simulink model "closedLoop_tuned"  (R2019a)
settings: Solver=ode14x  StartTime=0.0  StopTime=20  FixedStep=ts  RelTol=1e-3
undefined symbols (not defined in the file): ts
libraries: simulink x12, controlLibrary x12, mechLibrary x1
CloseFcn:
  | try,close(h1_elec_motor_brushless_dc),end
  | clear h1_elec_motor_brushless_dc
  | 
  | clear simlog_elec_motor_brushless_dc
  | clear logsout_elec_motor_brushless_dc
  | 
  | 
  | clear tout
Description:
  | Position feedback control, with servomotors, of a robot arm. Controllers are discretised.
  | 
  | Copyright 2008-2019 The MathWorks, Inc.
settings Model: DataDictionary=robotDataDictionary.sldd  EnableAccessToBaseWorkspace=off  Creator=MathWorks  LastModifiedBy=falderis
settings ConfigSet: Description=Configuration set for closed loop system
settings SolverCC: ExtrapolationOrder=1  SolverJacobianMethodControl=SparsePerturbation  AutoInsertRateTranBlk=on
settings DataIOCC: SaveFormat=StructureWithTime  SaveOutput=off  ReturnWorkspaceOutputsName=simulationOutput
settings OptimizationCC: BlockReduction=off  DefaultParameterBehavior=Inlined  EnhancedBackFolding=on  PassReuseOutputArgsAs=Individual arguments  OptimizeBlockOrder=speed  DifferentSizesBufferReuse=on  OptimizationCustomize=off
settings DebuggingCC: ParameterTunabilityLossMsg=error  BusObjectLabelMismatch=error  SFUnexpectedBacktrackingDiag=warning  SFNoUnconditionalDefaultTransitionDiag=warning  SFExecutionAtInitializationDiag=none  ArithmeticOperatorsInVariantConditions=warning
settings HardwareCC: ProdBitPerPointer=32  ProdBitPerSizeT=32  ProdBitPerPtrDiffT=32  ProdLargestAtomicFloat=None  ProdWordSize=32  ProdLongLongMode=on  ProdHWDeviceType=Generic->32-bit x86 compatible
settings ModelReferenceCC: ModelReferenceNumInstancesAllowed=Single  PropagateSignalLabelsOutOfModel=off
settings SFSimCC: SimUseLocalCustomCode=off  MATLABDynamicMemAlloc=off
settings RTWCC: SystemTargetFile=ert.tlc  TemplateMakefile=ert_default_tmf  GenerateReport=on  RTWVerbose=off  RTWUseLocalCustomCode=off  IncludeHyperlinkInReport=on  LaunchReport=on  CodeExecutionProfiling=on  GenerateTraceInfo=on  GenerateTraceReport=on  GenerateTraceReportSl=on  GenerateTraceReportSf=on  GenerateTraceReportEml=on  RTWCompilerOptimization=on
settings CodeAppCC: ForceParamTrailComments=on  IgnoreCustomStorageClasses=off  OperatorAnnotations=on  SimulinkDataObjDesc=on  SFDataObjDesc=on  InsertBlockDesc=on
settings ERTTargetCC: GenerateSampleERTMain=on  InlinedParameterPlacement=NonHierarchical  ERTCustomFileTemplate=example_file_process.tlc
settings ConfigComp: CovMetricSettings=dw  CovHtmlReporting=on  CovSaveCumulativeToWorkspaceVar=on  CovSaveSingleToWorkspaceVar=on  CovExternalEMLEnable=off  CovSFcnEnable=off
settings SimscapeCC: SimscapeNormalizeSystem=off  SimscapeLogName=mechPlant_simlog  SimscapeLogLimitData=off
settings ConfigurationSet: Description=SimMechanics 2G
settings ExplorerConfigSet: InternalSimMechanicsExplorerSettings="<ExplorerConfiguration><canonicalview>planar_xy</canonicalview><AnimationSetting><BasePlaybackSpeed>1.0</BasePlaybackSpeed><PlaybackSpeedFactor>1.0</PlaybackSpeedFactor></AnimationSetting><TilePanel><TileInfo><Tiles Columns=\"1\" Count=\"1\" Rows=\"1\"><Column Left=\"2\" Weight=\"1\"/><Column Left=\"833\"/><Row Top=\"2\" Weight=\"1\"/><Row Top=\"616\"/><Tile Height=\"1\" Width=\"1\" X=\"0\" Y=\"0\"/></Tiles></TileInfo><SceneInfo><SceneViewer><BGColor><R>0.60000002384185791</R><G>0.60000002384185791</G><B>0.60000002384185791</B></BGColor><Camera><Position><X>0.40313583982721529</X><Y>0.401665542364257</Y><Z>0.3417126092405493</Z></Position><Center><X>0.080205141109062281</X><Y>0.078734843646070099</Y><Z>0.018781910522366958</Z></Center><Up><X>-0.40824829046386307</X><Y>0.81649658092772615</Y><Z>-0.40824829046386307</Z></Up><Left>-0.31441769609555942</Left><Right>0.31441769609555942</Right><Bottom>-0.27755873043819368</Bottom><Top>0.27755873043819368</Top></Camera></SceneViewer></SceneInfo></TilePanel></ExplorerConfiguration>"

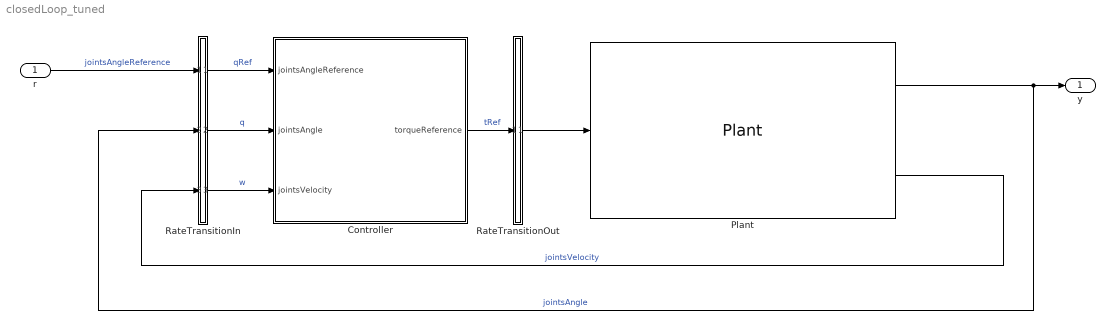
== system closedLoop_tuned ==
  r : Inport  OutDataTypeStr=Bus: jointMotionBus  Unit=deg  SampleTime=0
  Controller : Subsystem
      mask Display: image('controller.png')
  Plant : mechLibrary/Plant  SystemSampleTime=-1
  RateTransitionIn : Subsystem
  RateTransitionOut : Subsystem
  y : Outport  OutDataTypeStr=Bus: jointMotionBus  Unit=deg
  wires:
  Controller/1(torqueReference) -> RateTransitionOut/1(tRefIn)  "tRef"
  RateTransitionIn/1(qRef) -> Controller/1(jointsAngleReference)  "qRef"
  Plant/2 -> RateTransitionIn/3(wIn)  "jointsVelocity"
  RateTransitionOut/1(tRef) -> Plant/1
  RateTransitionIn/3(w) -> Controller/3(jointsVelocity)  "w"
  Plant/1 -> y/1, RateTransitionIn/2(qIn)  "jointsAngle"
  r/1 -> RateTransitionIn/1(qRefIn)  "jointsAngleReference"
  RateTransitionIn/2(q) -> Controller/2(jointsAngle)  "q"

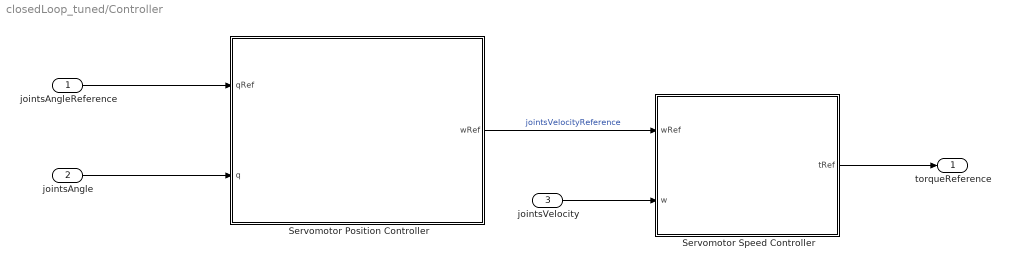
== system closedLoop_tuned/Controller ==
  jointsAngleReference : Inport  OutDataTypeStr=Bus: jointMotionBus  Unit=deg  SampleTime=ts
  jointsAngle : Inport  Port=2  OutDataTypeStr=Bus: jointMotionBus  Unit=deg  SampleTime=ts
  jointsVelocity : Inport  Port=3  OutDataTypeStr=Bus: jointVelBus  Unit=deg/s  SampleTime=ts
  Servomotor Position Controller : Subsystem  VariantControl=SV
      mask Display: image('pid.png');
  Servomotor Speed Controller : Subsystem
      mask Display: image('pi2.png');
  torqueReference : Outport  OutDataTypeStr=Bus: jointTorqueBus  Unit=N*m  SampleTime=ts
  wires:
  jointsAngle/1 -> Servomotor Position Controller/2(q)
  jointsAngleReference/1 -> Servomotor Position Controller/1(qRef)
  Servomotor Speed Controller/1(tRef) -> torqueReference/1
  Servomotor Position Controller/1(wRef) -> Servomotor Speed Controller/1(wRef)  "jointsVelocityReference"
  jointsVelocity/1 -> Servomotor Speed Controller/2(w)

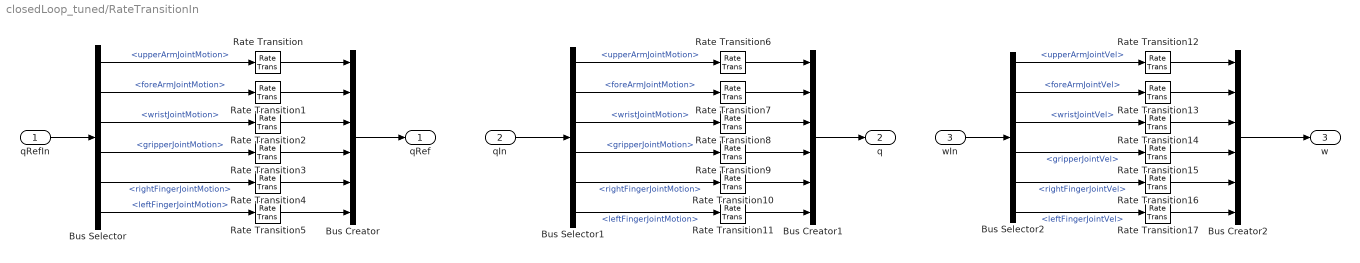
== system closedLoop_tuned/RateTransitionIn ==
  qRefIn : Inport  OutDataTypeStr=Bus: jointMotionBus  Unit=deg
  qIn : Inport  Port=2  OutDataTypeStr=Bus: jointMotionBus  Unit=deg
  wIn : Inport  Port=3  OutDataTypeStr=Bus: jointVelBus
  Bus Creator : BusCreator  Inputs=6  OutDataTypeStr=Bus: jointMotionBus
      settings: InheritFromInputs=off
  Bus Creator1 : BusCreator  Inputs=6  OutDataTypeStr=Bus: jointMotionBus
      settings: InheritFromInputs=off
  Bus Creator2 : BusCreator  Inputs=6  OutDataTypeStr=Bus: jointVelBus
      settings: InheritFromInputs=off
  Bus Selector : BusSelector  OutputSignals=upperArmJointMotion,foreArmJointMotion,wristJointMotion,gripperJointMotion,rightFingerJointMotion,leftFingerJointMotion
  Bus Selector1 : BusSelector  OutputSignals=upperArmJointMotion,foreArmJointMotion,wristJointMotion,gripperJointMotion,rightFingerJointMotion,leftFingerJointMotion
  Bus Selector2 : BusSelector  OutputSignals=upperArmJointVel,foreArmJointVel,wristJointVel,gripperJointVel,rightFingerJointVel,leftFingerJointVel
  Rate Transition{,1..17} (18 alike) : RateTransition  OutPortSampleTime=ts
  qRef : Outport  OutDataTypeStr=Bus: jointMotionBus
  q : Outport  Port=2  OutDataTypeStr=Bus: jointMotionBus
  w : Outport  Port=3  OutDataTypeStr=Bus: jointVelBus
  wires:
  Bus Selector1/6 -> Rate Transition11/1  "<leftFingerJointMotion>"
  Bus Selector1/3 -> Rate Transition8/1  "<wristJointMotion>"
  qIn/1 -> Bus Selector1/1
  Bus Selector1/1 -> Rate Transition6/1  "<upperArmJointMotion>"
  Bus Selector1/5 -> Rate Transition10/1  "<rightFingerJointMotion>"
  Bus Selector/6 -> Rate Transition5/1  "<leftFingerJointMotion>"
  Bus Selector1/4 -> Rate Transition9/1  "<gripperJointMotion>"
  Bus Selector/2 -> Rate Transition1/1  "<foreArmJointMotion>"
  Bus Selector1/2 -> Rate Transition7/1  "<foreArmJointMotion>"
  Bus Selector/3 -> Rate Transition2/1  "<wristJointMotion>"
  Bus Selector/4 -> Rate Transition3/1  "<gripperJointMotion>"
  Bus Selector/1 -> Rate Transition/1  "<upperArmJointMotion>"
  qRefIn/1 -> Bus Selector/1
  Bus Selector/5 -> Rate Transition4/1  "<rightFingerJointMotion>"
  Bus Selector2/5 -> Rate Transition16/1  "<rightFingerJointVel>"
  Bus Selector2/4 -> Rate Transition15/1  "<gripperJointVel>"
  Bus Selector2/3 -> Rate Transition14/1  "<wristJointVel>"
  wIn/1 -> Bus Selector2/1
  Bus Selector2/1 -> Rate Transition12/1  "<upperArmJointVel>"
  Bus Selector2/2 -> Rate Transition13/1  "<foreArmJointVel>"
  Bus Selector2/6 -> Rate Transition17/1  "<leftFingerJointVel>"
  Rate Transition/1 -> Bus Creator/1
  Rate Transition1/1 -> Bus Creator/2
  Rate Transition2/1 -> Bus Creator/3
  Rate Transition3/1 -> Bus Creator/4
  Rate Transition4/1 -> Bus Creator/5
  Rate Transition5/1 -> Bus Creator/6
  Bus Creator/1 -> qRef/1
  Rate Transition7/1 -> Bus Creator1/2
  Rate Transition11/1 -> Bus Creator1/6
  Bus Creator1/1 -> q/1
  Rate Transition9/1 -> Bus Creator1/4
  Rate Transition6/1 -> Bus Creator1/1
  Rate Transition8/1 -> Bus Creator1/3
  Rate Transition10/1 -> Bus Creator1/5
  Rate Transition12/1 -> Bus Creator2/1
  Rate Transition13/1 -> Bus Creator2/2
  Rate Transition14/1 -> Bus Creator2/3
  Rate Transition15/1 -> Bus Creator2/4
  Rate Transition16/1 -> Bus Creator2/5
  Rate Transition17/1 -> Bus Creator2/6
  Bus Creator2/1 -> w/1

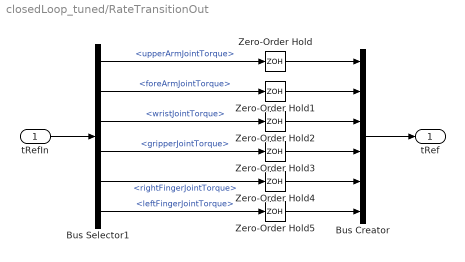
== system closedLoop_tuned/RateTransitionOut ==
  tRefIn : Inport  OutDataTypeStr=Bus: jointTorqueBus  Unit=N*m
  Bus Creator : BusCreator  Inputs=6  OutDataTypeStr=Bus: jointTorqueBus
      settings: InheritFromInputs=off
  Bus Selector1 : BusSelector  OutputSignals=upperArmJointTorque,foreArmJointTorque,wristJointTorque,gripperJointTorque,rightFingerJointTorque,leftFingerJointTorque
  Zero-Order Hold{,1..5} (6 alike) : ZeroOrderHold  SampleTime=-1
  tRef : Outport  OutDataTypeStr=Bus: jointTorqueBus  SampleTime=0
  wires:
  Bus Selector1/3 -> Zero-Order Hold2/1  "<wristJointTorque>"
  tRefIn/1 -> Bus Selector1/1
  Bus Selector1/2 -> Zero-Order Hold1/1  "<foreArmJointTorque>"
  Bus Selector1/5 -> Zero-Order Hold4/1  "<rightFingerJointTorque>"
  Bus Selector1/4 -> Zero-Order Hold3/1  "<gripperJointTorque>"
  Bus Selector1/1 -> Zero-Order Hold/1  "<upperArmJointTorque>"
  Bus Selector1/6 -> Zero-Order Hold5/1  "<leftFingerJointTorque>"
  Zero-Order Hold5/1 -> Bus Creator/6
  Zero-Order Hold4/1 -> Bus Creator/5
  Zero-Order Hold1/1 -> Bus Creator/2
  Zero-Order Hold/1 -> Bus Creator/1
  Zero-Order Hold2/1 -> Bus Creator/3
  Zero-Order Hold3/1 -> Bus Creator/4
  Bus Creator/1 -> tRef/1

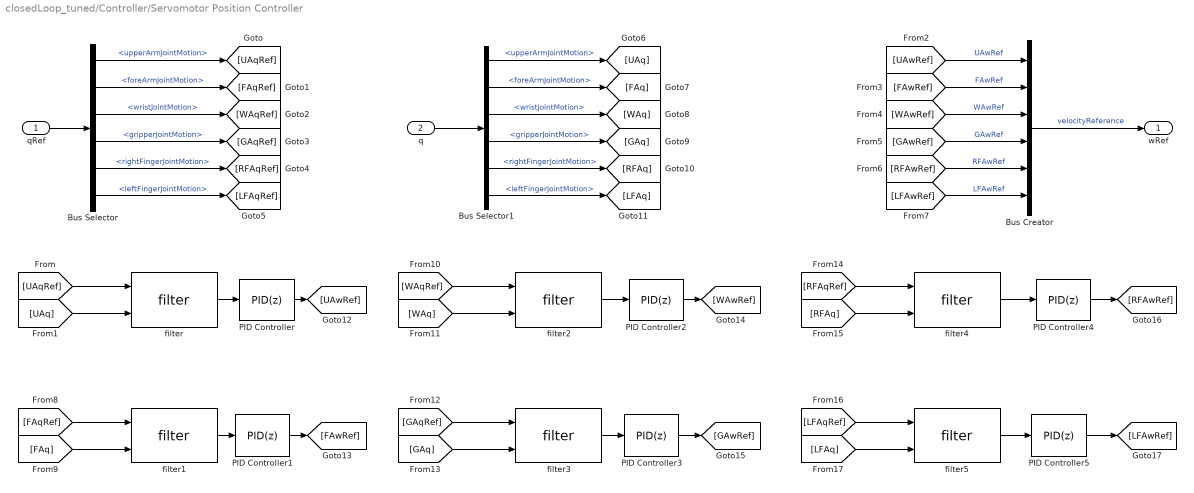
== system closedLoop_tuned/Controller/Servomotor Position Controller ==
  qRef : Inport  OutDataTypeStr=Bus: jointMotionBus  Unit=deg
  q : Inport  Port=2  OutDataTypeStr=Bus: jointMotionBus  Unit=deg
  Bus Creator : BusCreator  Inputs=6  OutDataTypeStr=Bus: jointVelBus
      settings: InheritFromInputs=off
  Bus Selector : BusSelector  OutputSignals=upperArmJointMotion,foreArmJointMotion,wristJointMotion,gripperJointMotion,rightFingerJointMotion,leftFingerJointMotion
  Bus Selector1 : BusSelector  OutputSignals=upperArmJointMotion,foreArmJointMotion,wristJointMotion,gripperJointMotion,rightFingerJointMotion,leftFingerJointMotion
  PID Controller : simulink/Continuous/PID Controller  Controller=PID  Form=Parallel  TimeDomain=Discrete-time  SampleTime=ts  IntegratorMethod=Forward Euler  FilterMethod=Forward Euler  ControllerParametersSource=internal  P=10.4708336285486  I=0.000419222702982036  D=0.346600752490046  UseFilter=on  N=761.904761904762  TunerSelectOption=Transfer Function Based (PID Tuner App)  InitialConditionSource=internal  InitialConditionForIntegrator=0  InitialConditionForFilter=0  DifferentiatorICPrevScaledInput=0  ExternalReset=none  TrackingMode=off  Kt=1  LimitOutput=off  UpperSaturationLimit=inf  LowerSaturationLimit=-inf  LinearizeAsGain=on  AntiWindupMode=none  Kb=1  POutMin=[]  POutMax=[]  IOutMin=[]  IOutMax=[]  DOutMin=[]  DOutMax=[]  NOutMin=[]  NOutMax=[]  SumOutMin=[]  SumOutMax=[]  SaturationOutMin=[]  SaturationOutMax=[]  PParamMin=[]  PParamMax=[]  IParamMin=[]  IParamMax=[]  DParamMin=[]  DParamMax=[]  NParamMin=[]  NParamMax=[]  KbParamMin=[]  KbParamMax=[]  KtParamMin=[]  KtParamMax=[]  KbOutMin=[]  KbOutMax=[]  KtOutMin=[]  KtOutMax=[]  IntegratorOutMin=[]  IntegratorOutMax=[]  FilterOutMin=[]  FilterOutMax=[]  SumI1OutMin=[]  SumI1OutMax=[]  SumI2OutMin=[]  SumI2OutMax=[]  SumI3OutMin=[]  SumI3OutMax=[]  SumI4OutMin=[]  SumI4OutMax=[]  SumDOutMin=[]  SumDOutMax=[]  DifferentiatorOutMin=[]  DifferentiatorOutMax=[]  FilterDiffOutCoefMin=[]  FilterDiffOutCoefMax=[]  ReciprocalOutMin=[]  ReciprocalOutMax=[]  SumDenOutMin=[]  SumDenOutMax=[]  SumNumOutMin=[]  SumNumOutMax=[]  DivideOutMin=[]  DivideOutMax=[]  IntegratorContinuousStateAttributes=''  IntegratorStateMustResolveToSignalObject=off  IntegratorRTWStateStorageClass=Auto  FilterContinuousStateAttributes=''  FilterStateMustResolveToSignalObject=off  FilterRTWStateStorageClass=Auto  ParallelPVariant=InternalParameters  IdealPVariant=Disabled  IVariant=InternalParameters  DVariant=InternalParameters  IntegratorVariant=Discrete  SatVariant=Disabled  AWVariant=Passthrough  PCopyVariant=Disabled  TRVariant=Disabled  FdbkBlocksVariant=Forward  IdealPFdbkVariant=Disabled  SatFdbkVariant=Disabled  DerivativeFilterVariant=ForwardEulerFilter  NVariant=InternalParameters  NCopyVariant=Disabled  FilterICVariant=InternalICsFilter  IntegratorICVariant=InternalICs  ExternalResetVariant=Disabled  TRSumVariant=Passthrough  SumFdbkVariant=Disabled  SumVariant=Sum_PID
  PID Controller1 : simulink/Continuous/PID Controller  Controller=PID  Form=Parallel  TimeDomain=Discrete-time  SampleTime=ts  IntegratorMethod=Forward Euler  FilterMethod=Forward Euler  ControllerParametersSource=internal  P=10.7694124560307  I=0.000593032145468798  D=21.0180234727249  UseFilter=on  N=4.00240654506278e-05  TunerSelectOption=Transfer Function Based (PID Tuner App)  InitialConditionSource=internal  InitialConditionForIntegrator=0  InitialConditionForFilter=0  DifferentiatorICPrevScaledInput=0  ExternalReset=none  TrackingMode=off  Kt=1  LimitOutput=off  UpperSaturationLimit=inf  LowerSaturationLimit=-inf  LinearizeAsGain=on  AntiWindupMode=none  Kb=1  POutMin=[]  POutMax=[]  IOutMin=[]  IOutMax=[]  DOutMin=[]  DOutMax=[]  NOutMin=[]  NOutMax=[]  SumOutMin=[]  SumOutMax=[]  SaturationOutMin=[]  SaturationOutMax=[]  PParamMin=[]  PParamMax=[]  IParamMin=[]  IParamMax=[]  DParamMin=[]  DParamMax=[]  NParamMin=[]  NParamMax=[]  KbParamMin=[]  KbParamMax=[]  KtParamMin=[]  KtParamMax=[]  KbOutMin=[]  KbOutMax=[]  KtOutMin=[]  KtOutMax=[]  IntegratorOutMin=[]  IntegratorOutMax=[]  FilterOutMin=[]  FilterOutMax=[]  SumI1OutMin=[]  SumI1OutMax=[]  SumI2OutMin=[]  SumI2OutMax=[]  SumI3OutMin=[]  SumI3OutMax=[]  SumI4OutMin=[]  SumI4OutMax=[]  SumDOutMin=[]  SumDOutMax=[]  DifferentiatorOutMin=[]  DifferentiatorOutMax=[]  FilterDiffOutCoefMin=[]  FilterDiffOutCoefMax=[]  ReciprocalOutMin=[]  ReciprocalOutMax=[]  SumDenOutMin=[]  SumDenOutMax=[]  SumNumOutMin=[]  SumNumOutMax=[]  DivideOutMin=[]  DivideOutMax=[]  IntegratorContinuousStateAttributes=''  IntegratorStateMustResolveToSignalObject=off  IntegratorRTWStateStorageClass=Auto  FilterContinuousStateAttributes=''  FilterStateMustResolveToSignalObject=off  FilterRTWStateStorageClass=Auto  ParallelPVariant=InternalParameters  IdealPVariant=Disabled  IVariant=InternalParameters  DVariant=InternalParameters  IntegratorVariant=Discrete  SatVariant=Disabled  AWVariant=Passthrough  PCopyVariant=Disabled  TRVariant=Disabled  FdbkBlocksVariant=Forward  IdealPFdbkVariant=Disabled  SatFdbkVariant=Disabled  DerivativeFilterVariant=ForwardEulerFilter  NVariant=InternalParameters  NCopyVariant=Disabled  FilterICVariant=InternalICsFilter  IntegratorICVariant=InternalICs  ExternalResetVariant=Disabled  TRSumVariant=Passthrough  SumFdbkVariant=Disabled  SumVariant=Sum_PID
  PID Controller2 : simulink/Continuous/PID Controller  Controller=PID  Form=Parallel  TimeDomain=Discrete-time  SampleTime=ts  IntegratorMethod=Forward Euler  FilterMethod=Forward Euler  ControllerParametersSource=internal  P=10.8442867281081  I=0.000448190430142682  D=0.223470955257761  UseFilter=on  N=761.904761904762  TunerSelectOption=Transfer Function Based (PID Tuner App)  InitialConditionSource=internal  InitialConditionForIntegrator=0  InitialConditionForFilter=0  DifferentiatorICPrevScaledInput=0  ExternalReset=none  TrackingMode=off  Kt=1  LimitOutput=off  UpperSaturationLimit=inf  LowerSaturationLimit=-inf  LinearizeAsGain=on  AntiWindupMode=none  Kb=1  POutMin=[]  POutMax=[]  IOutMin=[]  IOutMax=[]  DOutMin=[]  DOutMax=[]  NOutMin=[]  NOutMax=[]  SumOutMin=[]  SumOutMax=[]  SaturationOutMin=[]  SaturationOutMax=[]  PParamMin=[]  PParamMax=[]  IParamMin=[]  IParamMax=[]  DParamMin=[]  DParamMax=[]  NParamMin=[]  NParamMax=[]  KbParamMin=[]  KbParamMax=[]  KtParamMin=[]  KtParamMax=[]  KbOutMin=[]  KbOutMax=[]  KtOutMin=[]  KtOutMax=[]  IntegratorOutMin=[]  IntegratorOutMax=[]  FilterOutMin=[]  FilterOutMax=[]  SumI1OutMin=[]  SumI1OutMax=[]  SumI2OutMin=[]  SumI2OutMax=[]  SumI3OutMin=[]  SumI3OutMax=[]  SumI4OutMin=[]  SumI4OutMax=[]  SumDOutMin=[]  SumDOutMax=[]  DifferentiatorOutMin=[]  DifferentiatorOutMax=[]  FilterDiffOutCoefMin=[]  FilterDiffOutCoefMax=[]  ReciprocalOutMin=[]  ReciprocalOutMax=[]  SumDenOutMin=[]  SumDenOutMax=[]  SumNumOutMin=[]  SumNumOutMax=[]  DivideOutMin=[]  DivideOutMax=[]  IntegratorContinuousStateAttributes=''  IntegratorStateMustResolveToSignalObject=off  IntegratorRTWStateStorageClass=Auto  FilterContinuousStateAttributes=''  FilterStateMustResolveToSignalObject=off  FilterRTWStateStorageClass=Auto  ParallelPVariant=InternalParameters  IdealPVariant=Disabled  IVariant=InternalParameters  DVariant=InternalParameters  IntegratorVariant=Discrete  SatVariant=Disabled  AWVariant=Passthrough  PCopyVariant=Disabled  TRVariant=Disabled  FdbkBlocksVariant=Forward  IdealPFdbkVariant=Disabled  SatFdbkVariant=Disabled  DerivativeFilterVariant=ForwardEulerFilter  NVariant=InternalParameters  NCopyVariant=Disabled  FilterICVariant=InternalICsFilter  IntegratorICVariant=InternalICs  ExternalResetVariant=Disabled  TRSumVariant=Passthrough  SumFdbkVariant=Disabled  SumVariant=Sum_PID
  PID Controller3 : simulink/Continuous/PID Controller  Controller=PID  Form=Parallel  TimeDomain=Discrete-time  SampleTime=ts  IntegratorMethod=Forward Euler  FilterMethod=Forward Euler  ControllerParametersSource=internal  P=9.66802754702183  I=0.000444755466308859  D=58.2762205966547  UseFilter=on  N=0.0216415897548656  TunerSelectOption=Transfer Function Based (PID Tuner App)  InitialConditionSource=internal  InitialConditionForIntegrator=0  InitialConditionForFilter=0  DifferentiatorICPrevScaledInput=0  ExternalReset=none  TrackingMode=off  Kt=1  LimitOutput=off  UpperSaturationLimit=inf  LowerSaturationLimit=-inf  LinearizeAsGain=on  AntiWindupMode=none  Kb=1  POutMin=[]  POutMax=[]  IOutMin=[]  IOutMax=[]  DOutMin=[]  DOutMax=[]  NOutMin=[]  NOutMax=[]  SumOutMin=[]  SumOutMax=[]  SaturationOutMin=[]  SaturationOutMax=[]  PParamMin=[]  PParamMax=[]  IParamMin=[]  IParamMax=[]  DParamMin=[]  DParamMax=[]  NParamMin=[]  NParamMax=[]  KbParamMin=[]  KbParamMax=[]  KtParamMin=[]  KtParamMax=[]  KbOutMin=[]  KbOutMax=[]  KtOutMin=[]  KtOutMax=[]  IntegratorOutMin=[]  IntegratorOutMax=[]  FilterOutMin=[]  FilterOutMax=[]  SumI1OutMin=[]  SumI1OutMax=[]  SumI2OutMin=[]  SumI2OutMax=[]  SumI3OutMin=[]  SumI3OutMax=[]  SumI4OutMin=[]  SumI4OutMax=[]  SumDOutMin=[]  SumDOutMax=[]  DifferentiatorOutMin=[]  DifferentiatorOutMax=[]  FilterDiffOutCoefMin=[]  FilterDiffOutCoefMax=[]  ReciprocalOutMin=[]  ReciprocalOutMax=[]  SumDenOutMin=[]  SumDenOutMax=[]  SumNumOutMin=[]  SumNumOutMax=[]  DivideOutMin=[]  DivideOutMax=[]  IntegratorContinuousStateAttributes=''  IntegratorStateMustResolveToSignalObject=off  IntegratorRTWStateStorageClass=Auto  FilterContinuousStateAttributes=''  FilterStateMustResolveToSignalObject=off  FilterRTWStateStorageClass=Auto  ParallelPVariant=InternalParameters  IdealPVariant=Disabled  IVariant=InternalParameters  DVariant=InternalParameters  IntegratorVariant=Discrete  SatVariant=Disabled  AWVariant=Passthrough  PCopyVariant=Disabled  TRVariant=Disabled  FdbkBlocksVariant=Forward  IdealPFdbkVariant=Disabled  SatFdbkVariant=Disabled  DerivativeFilterVariant=ForwardEulerFilter  NVariant=InternalParameters  NCopyVariant=Disabled  FilterICVariant=InternalICsFilter  IntegratorICVariant=InternalICs  ExternalResetVariant=Disabled  TRSumVariant=Passthrough  SumFdbkVariant=Disabled  SumVariant=Sum_PID
  PID Controller4 : simulink/Continuous/PID Controller  Controller=PID  Form=Parallel  TimeDomain=Discrete-time  SampleTime=ts  IntegratorMethod=Forward Euler  FilterMethod=Forward Euler  ControllerParametersSource=internal  P=10.7702769040942  I=0.00097597573827831  D=0.195709489924621  UseFilter=on  N=190.172011630327  TunerSelectOption=Transfer Function Based (PID Tuner App)  InitialConditionSource=internal  InitialConditionForIntegrator=0  InitialConditionForFilter=0  DifferentiatorICPrevScaledInput=0  ExternalReset=none  TrackingMode=off  Kt=1  LimitOutput=off  UpperSaturationLimit=inf  LowerSaturationLimit=-inf  LinearizeAsGain=on  AntiWindupMode=none  Kb=1  POutMin=[]  POutMax=[]  IOutMin=[]  IOutMax=[]  DOutMin=[]  DOutMax=[]  NOutMin=[]  NOutMax=[]  SumOutMin=[]  SumOutMax=[]  SaturationOutMin=[]  SaturationOutMax=[]  PParamMin=[]  PParamMax=[]  IParamMin=[]  IParamMax=[]  DParamMin=[]  DParamMax=[]  NParamMin=[]  NParamMax=[]  KbParamMin=[]  KbParamMax=[]  KtParamMin=[]  KtParamMax=[]  KbOutMin=[]  KbOutMax=[]  KtOutMin=[]  KtOutMax=[]  IntegratorOutMin=[]  IntegratorOutMax=[]  FilterOutMin=[]  FilterOutMax=[]  SumI1OutMin=[]  SumI1OutMax=[]  SumI2OutMin=[]  SumI2OutMax=[]  SumI3OutMin=[]  SumI3OutMax=[]  SumI4OutMin=[]  SumI4OutMax=[]  SumDOutMin=[]  SumDOutMax=[]  DifferentiatorOutMin=[]  DifferentiatorOutMax=[]  FilterDiffOutCoefMin=[]  FilterDiffOutCoefMax=[]  ReciprocalOutMin=[]  ReciprocalOutMax=[]  SumDenOutMin=[]  SumDenOutMax=[]  SumNumOutMin=[]  SumNumOutMax=[]  DivideOutMin=[]  DivideOutMax=[]  IntegratorContinuousStateAttributes=''  IntegratorStateMustResolveToSignalObject=off  IntegratorRTWStateStorageClass=Auto  FilterContinuousStateAttributes=''  FilterStateMustResolveToSignalObject=off  FilterRTWStateStorageClass=Auto  ParallelPVariant=InternalParameters  IdealPVariant=Disabled  IVariant=InternalParameters  DVariant=InternalParameters  IntegratorVariant=Discrete  SatVariant=Disabled  AWVariant=Passthrough  PCopyVariant=Disabled  TRVariant=Disabled  FdbkBlocksVariant=Forward  IdealPFdbkVariant=Disabled  SatFdbkVariant=Disabled  DerivativeFilterVariant=ForwardEulerFilter  NVariant=InternalParameters  NCopyVariant=Disabled  FilterICVariant=InternalICsFilter  IntegratorICVariant=InternalICs  ExternalResetVariant=Disabled  TRSumVariant=Passthrough  SumFdbkVariant=Disabled  SumVariant=Sum_PID
  PID Controller5 : simulink/Continuous/PID Controller  Controller=PID  Form=Parallel  TimeDomain=Discrete-time  SampleTime=ts  IntegratorMethod=Forward Euler  FilterMethod=Forward Euler  ControllerParametersSource=internal  P=10.7654470599538  I=0.00114163073091871  D=0.20047626148189  UseFilter=on  N=257.755378801474  TunerSelectOption=Transfer Function Based (PID Tuner App)  InitialConditionSource=internal  InitialConditionForIntegrator=0  InitialConditionForFilter=0  DifferentiatorICPrevScaledInput=0  ExternalReset=none  TrackingMode=off  Kt=1  LimitOutput=off  UpperSaturationLimit=inf  LowerSaturationLimit=-inf  LinearizeAsGain=on  AntiWindupMode=none  Kb=1  POutMin=[]  POutMax=[]  IOutMin=[]  IOutMax=[]  DOutMin=[]  DOutMax=[]  NOutMin=[]  NOutMax=[]  SumOutMin=[]  SumOutMax=[]  SaturationOutMin=[]  SaturationOutMax=[]  PParamMin=[]  PParamMax=[]  IParamMin=[]  IParamMax=[]  DParamMin=[]  DParamMax=[]  NParamMin=[]  NParamMax=[]  KbParamMin=[]  KbParamMax=[]  KtParamMin=[]  KtParamMax=[]  KbOutMin=[]  KbOutMax=[]  KtOutMin=[]  KtOutMax=[]  IntegratorOutMin=[]  IntegratorOutMax=[]  FilterOutMin=[]  FilterOutMax=[]  SumI1OutMin=[]  SumI1OutMax=[]  SumI2OutMin=[]  SumI2OutMax=[]  SumI3OutMin=[]  SumI3OutMax=[]  SumI4OutMin=[]  SumI4OutMax=[]  SumDOutMin=[]  SumDOutMax=[]  DifferentiatorOutMin=[]  DifferentiatorOutMax=[]  FilterDiffOutCoefMin=[]  FilterDiffOutCoefMax=[]  ReciprocalOutMin=[]  ReciprocalOutMax=[]  SumDenOutMin=[]  SumDenOutMax=[]  SumNumOutMin=[]  SumNumOutMax=[]  DivideOutMin=[]  DivideOutMax=[]  IntegratorContinuousStateAttributes=''  IntegratorStateMustResolveToSignalObject=off  IntegratorRTWStateStorageClass=Auto  FilterContinuousStateAttributes=''  FilterStateMustResolveToSignalObject=off  FilterRTWStateStorageClass=Auto  ParallelPVariant=InternalParameters  IdealPVariant=Disabled  IVariant=InternalParameters  DVariant=InternalParameters  IntegratorVariant=Discrete  SatVariant=Disabled  AWVariant=Passthrough  PCopyVariant=Disabled  TRVariant=Disabled  FdbkBlocksVariant=Forward  IdealPFdbkVariant=Disabled  SatFdbkVariant=Disabled  DerivativeFilterVariant=ForwardEulerFilter  NVariant=InternalParameters  NCopyVariant=Disabled  FilterICVariant=InternalICsFilter  IntegratorICVariant=InternalICs  ExternalResetVariant=Disabled  TRSumVariant=Passthrough  SumFdbkVariant=Disabled  SumVariant=Sum_PID
  filter{,1..5} (6 alike) : controlLibrary/filter  tc=1e-2  sampleTime=ts
  wRef : Outport  OutDataTypeStr=Bus: jointVelBus  Unit=deg/s
  wires:
  qRef/1 -> Bus Selector/1
  q/1 -> Bus Selector1/1
  Bus Selector/1 -> [UAqRef]  "<upperArmJointMotion>"
  Bus Selector/2 -> [FAqRef]  "<foreArmJointMotion>"
  Bus Selector/3 -> [WAqRef]  "<wristJointMotion>"
  Bus Selector/4 -> [GAqRef]  "<gripperJointMotion>"
  Bus Selector/5 -> [RFAqRef]  "<rightFingerJointMotion>"
  Bus Selector/6 -> [LFAqRef]  "<leftFingerJointMotion>"
  Bus Selector1/1 -> [UAq]  "<upperArmJointMotion>"
  Bus Selector1/3 -> [WAq]  "<wristJointMotion>"
  Bus Selector1/2 -> [FAq]  "<foreArmJointMotion>"
  Bus Selector1/5 -> [RFAq]  "<rightFingerJointMotion>"
  Bus Selector1/4 -> [GAq]  "<gripperJointMotion>"
  Bus Selector1/6 -> [LFAq]  "<leftFingerJointMotion>"
  [UAwRef] -> Bus Creator/1  "UAwRef"
  [FAwRef] -> Bus Creator/2  "FAwRef"
  [WAwRef] -> Bus Creator/3  "WAwRef"
  [GAwRef] -> Bus Creator/4  "GAwRef"
  [RFAwRef] -> Bus Creator/5  "RFAwRef"
  [LFAwRef] -> Bus Creator/6  "LFAwRef"
  Bus Creator/1 -> wRef/1  "velocityReference"
  filter5/1 -> PID Controller5/1
  [RFAq] -> filter4/2
  [LFAq] -> filter5/2
  [FAqRef] -> filter1/1
  [GAqRef] -> filter3/1
  filter3/1 -> PID Controller3/1
  [UAq] -> filter/2
  [RFAqRef] -> filter4/1
  [WAq] -> filter2/2
  [UAqRef] -> filter/1
  filter2/1 -> PID Controller2/1
  [WAqRef] -> filter2/1
  [FAq] -> filter1/2
  [GAq] -> filter3/2
  [LFAqRef] -> filter5/1
  filter4/1 -> PID Controller4/1
  filter/1 -> PID Controller/1
  PID Controller/1 -> [UAwRef]
  PID Controller2/1 -> [WAwRef]
  PID Controller3/1 -> [GAwRef]
  PID Controller4/1 -> [RFAwRef]
  PID Controller5/1 -> [LFAwRef]
  filter1/1 -> PID Controller1/1
  PID Controller1/1 -> [FAwRef]

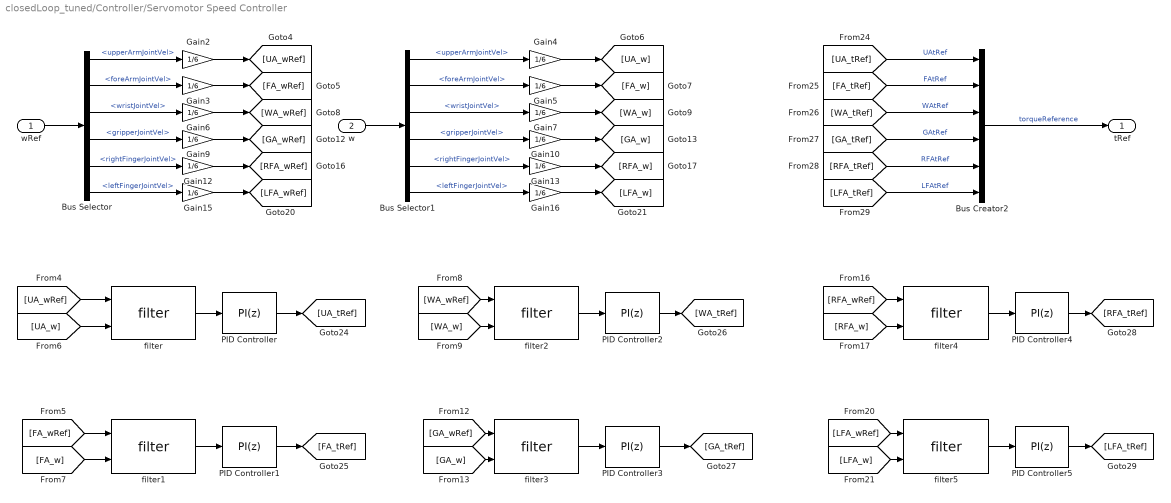
== system closedLoop_tuned/Controller/Servomotor Speed Controller ==
  wRef : Inport  OutDataTypeStr=Bus: jointVelBus
  w : Inport  Port=2  OutDataTypeStr=Bus: jointVelBus
  Bus Creator2 : BusCreator  Inputs=6  OutDataTypeStr=Bus: jointTorqueBus
      settings: InheritFromInputs=off
  Bus Selector : BusSelector  OutputSignals=upperArmJointVel,foreArmJointVel,wristJointVel,gripperJointVel,rightFingerJointVel,leftFingerJointVel
  Bus Selector1 : BusSelector  OutputSignals=upperArmJointVel,foreArmJointVel,wristJointVel,gripperJointVel,rightFingerJointVel,leftFingerJointVel
  Gain{2..7,9..10,12..13,15..16} (12 alike) : Gain  Gain=1/6
  PID Controller : simulink/Continuous/PID Controller  Controller=PI  Form=Parallel  TimeDomain=Discrete-time  SampleTime=ts  IntegratorMethod=Forward Euler  FilterMethod=Forward Euler  ControllerParametersSource=internal  P=0.0360231984902585  I=0.00337174988064101  D=0  UseFilter=on  N=0  TunerSelectOption=Transfer Function Based (PID Tuner App)  InitialConditionSource=internal  InitialConditionForIntegrator=0  InitialConditionForFilter=0  DifferentiatorICPrevScaledInput=0  ExternalReset=none  TrackingMode=off  Kt=1  LimitOutput=off  UpperSaturationLimit=inf  LowerSaturationLimit=-inf  LinearizeAsGain=on  AntiWindupMode=none  Kb=1  POutMin=[]  POutMax=[]  IOutMin=[]  IOutMax=[]  DOutMin=[]  DOutMax=[]  NOutMin=[]  NOutMax=[]  SumOutMin=[]  SumOutMax=[]  SaturationOutMin=[]  SaturationOutMax=[]  PParamMin=[]  PParamMax=[]  IParamMin=[]  IParamMax=[]  DParamMin=[]  DParamMax=[]  NParamMin=[]  NParamMax=[]  KbParamMin=[]  KbParamMax=[]  KtParamMin=[]  KtParamMax=[]  KbOutMin=[]  KbOutMax=[]  KtOutMin=[]  KtOutMax=[]  IntegratorOutMin=[]  IntegratorOutMax=[]  FilterOutMin=[]  FilterOutMax=[]  SumI1OutMin=[]  SumI1OutMax=[]  SumI2OutMin=[]  SumI2OutMax=[]  SumI3OutMin=[]  SumI3OutMax=[]  SumI4OutMin=[]  SumI4OutMax=[]  SumDOutMin=[]  SumDOutMax=[]  DifferentiatorOutMin=[]  DifferentiatorOutMax=[]  FilterDiffOutCoefMin=[]  FilterDiffOutCoefMax=[]  ReciprocalOutMin=[]  ReciprocalOutMax=[]  SumDenOutMin=[]  SumDenOutMax=[]  SumNumOutMin=[]  SumNumOutMax=[]  DivideOutMin=[]  DivideOutMax=[]  IntegratorContinuousStateAttributes=''  IntegratorStateMustResolveToSignalObject=off  IntegratorRTWStateStorageClass=Auto  FilterContinuousStateAttributes=''  FilterStateMustResolveToSignalObject=off  FilterRTWStateStorageClass=Auto  ParallelPVariant=InternalParameters  IdealPVariant=Disabled  IVariant=InternalParameters  DVariant=Disabled  IntegratorVariant=Discrete  SatVariant=Disabled  AWVariant=Passthrough  PCopyVariant=Disabled  TRVariant=Disabled  FdbkBlocksVariant=Forward  IdealPFdbkVariant=Disabled  SatFdbkVariant=Disabled  DerivativeFilterVariant=Disabled  NVariant=Disabled  NCopyVariant=Disabled_SignalSpec  FilterICVariant=Disabled  IntegratorICVariant=InternalICs  ExternalResetVariant=Disabled  TRSumVariant=Passthrough  SumFdbkVariant=Disabled  SumVariant=Sum_PI
  PID Controller1 : simulink/Continuous/PID Controller  Controller=PI  Form=Parallel  TimeDomain=Discrete-time  SampleTime=ts  IntegratorMethod=Forward Euler  FilterMethod=Forward Euler  ControllerParametersSource=internal  P=0.0192799899284329  I=2.06091269945642  D=0  UseFilter=on  N=0  TunerSelectOption=Transfer Function Based (PID Tuner App)  InitialConditionSource=internal  InitialConditionForIntegrator=0  InitialConditionForFilter=0  DifferentiatorICPrevScaledInput=0  ExternalReset=none  TrackingMode=off  Kt=1  LimitOutput=off  UpperSaturationLimit=inf  LowerSaturationLimit=-inf  LinearizeAsGain=on  AntiWindupMode=none  Kb=1  POutMin=[]  POutMax=[]  IOutMin=[]  IOutMax=[]  DOutMin=[]  DOutMax=[]  NOutMin=[]  NOutMax=[]  SumOutMin=[]  SumOutMax=[]  SaturationOutMin=[]  SaturationOutMax=[]  PParamMin=[]  PParamMax=[]  IParamMin=[]  IParamMax=[]  DParamMin=[]  DParamMax=[]  NParamMin=[]  NParamMax=[]  KbParamMin=[]  KbParamMax=[]  KtParamMin=[]  KtParamMax=[]  KbOutMin=[]  KbOutMax=[]  KtOutMin=[]  KtOutMax=[]  IntegratorOutMin=[]  IntegratorOutMax=[]  FilterOutMin=[]  FilterOutMax=[]  SumI1OutMin=[]  SumI1OutMax=[]  SumI2OutMin=[]  SumI2OutMax=[]  SumI3OutMin=[]  SumI3OutMax=[]  SumI4OutMin=[]  SumI4OutMax=[]  SumDOutMin=[]  SumDOutMax=[]  DifferentiatorOutMin=[]  DifferentiatorOutMax=[]  FilterDiffOutCoefMin=[]  FilterDiffOutCoefMax=[]  ReciprocalOutMin=[]  ReciprocalOutMax=[]  SumDenOutMin=[]  SumDenOutMax=[]  SumNumOutMin=[]  SumNumOutMax=[]  DivideOutMin=[]  DivideOutMax=[]  IntegratorContinuousStateAttributes=''  IntegratorStateMustResolveToSignalObject=off  IntegratorRTWStateStorageClass=Auto  FilterContinuousStateAttributes=''  FilterStateMustResolveToSignalObject=off  FilterRTWStateStorageClass=Auto  ParallelPVariant=InternalParameters  IdealPVariant=Disabled  IVariant=InternalParameters  DVariant=Disabled  IntegratorVariant=Discrete  SatVariant=Disabled  AWVariant=Passthrough  PCopyVariant=Disabled  TRVariant=Disabled  FdbkBlocksVariant=Forward  IdealPFdbkVariant=Disabled  SatFdbkVariant=Disabled  DerivativeFilterVariant=Disabled  NVariant=Disabled  NCopyVariant=Disabled_SignalSpec  FilterICVariant=Disabled  IntegratorICVariant=InternalICs  ExternalResetVariant=Disabled  TRSumVariant=Passthrough  SumFdbkVariant=Disabled  SumVariant=Sum_PI
  PID Controller2 : simulink/Continuous/PID Controller  Controller=PI  Form=Parallel  TimeDomain=Discrete-time  SampleTime=ts  IntegratorMethod=Forward Euler  FilterMethod=Forward Euler  ControllerParametersSource=internal  P=0.0426832255455665  I=0.0265288646840578  D=0  UseFilter=on  N=0  TunerSelectOption=Transfer Function Based (PID Tuner App)  InitialConditionSource=internal  InitialConditionForIntegrator=0  InitialConditionForFilter=0  DifferentiatorICPrevScaledInput=0  ExternalReset=none  TrackingMode=off  Kt=1  LimitOutput=off  UpperSaturationLimit=inf  LowerSaturationLimit=-inf  LinearizeAsGain=on  AntiWindupMode=none  Kb=1  POutMin=[]  POutMax=[]  IOutMin=[]  IOutMax=[]  DOutMin=[]  DOutMax=[]  NOutMin=[]  NOutMax=[]  SumOutMin=[]  SumOutMax=[]  SaturationOutMin=[]  SaturationOutMax=[]  PParamMin=[]  PParamMax=[]  IParamMin=[]  IParamMax=[]  DParamMin=[]  DParamMax=[]  NParamMin=[]  NParamMax=[]  KbParamMin=[]  KbParamMax=[]  KtParamMin=[]  KtParamMax=[]  KbOutMin=[]  KbOutMax=[]  KtOutMin=[]  KtOutMax=[]  IntegratorOutMin=[]  IntegratorOutMax=[]  FilterOutMin=[]  FilterOutMax=[]  SumI1OutMin=[]  SumI1OutMax=[]  SumI2OutMin=[]  SumI2OutMax=[]  SumI3OutMin=[]  SumI3OutMax=[]  SumI4OutMin=[]  SumI4OutMax=[]  SumDOutMin=[]  SumDOutMax=[]  DifferentiatorOutMin=[]  DifferentiatorOutMax=[]  FilterDiffOutCoefMin=[]  FilterDiffOutCoefMax=[]  ReciprocalOutMin=[]  ReciprocalOutMax=[]  SumDenOutMin=[]  SumDenOutMax=[]  SumNumOutMin=[]  SumNumOutMax=[]  DivideOutMin=[]  DivideOutMax=[]  IntegratorContinuousStateAttributes=''  IntegratorStateMustResolveToSignalObject=off  IntegratorRTWStateStorageClass=Auto  FilterContinuousStateAttributes=''  FilterStateMustResolveToSignalObject=off  FilterRTWStateStorageClass=Auto  ParallelPVariant=InternalParameters  IdealPVariant=Disabled  IVariant=InternalParameters  DVariant=Disabled  IntegratorVariant=Discrete  SatVariant=Disabled  AWVariant=Passthrough  PCopyVariant=Disabled  TRVariant=Disabled  FdbkBlocksVariant=Forward  IdealPFdbkVariant=Disabled  SatFdbkVariant=Disabled  DerivativeFilterVariant=Disabled  NVariant=Disabled  NCopyVariant=Disabled_SignalSpec  FilterICVariant=Disabled  IntegratorICVariant=InternalICs  ExternalResetVariant=Disabled  TRSumVariant=Passthrough  SumFdbkVariant=Disabled  SumVariant=Sum_PI
  PID Controller3 : simulink/Continuous/PID Controller  Controller=PI  Form=Parallel  TimeDomain=Discrete-time  SampleTime=ts  IntegratorMethod=Forward Euler  FilterMethod=Forward Euler  ControllerParametersSource=internal  P=0.00572339896932079  I=0.460092048608168  D=0  UseFilter=on  N=0  TunerSelectOption=Transfer Function Based (PID Tuner App)  InitialConditionSource=internal  InitialConditionForIntegrator=0  InitialConditionForFilter=0  DifferentiatorICPrevScaledInput=0  ExternalReset=none  TrackingMode=off  Kt=1  LimitOutput=off  UpperSaturationLimit=inf  LowerSaturationLimit=-inf  LinearizeAsGain=on  AntiWindupMode=none  Kb=1  POutMin=[]  POutMax=[]  IOutMin=[]  IOutMax=[]  DOutMin=[]  DOutMax=[]  NOutMin=[]  NOutMax=[]  SumOutMin=[]  SumOutMax=[]  SaturationOutMin=[]  SaturationOutMax=[]  PParamMin=[]  PParamMax=[]  IParamMin=[]  IParamMax=[]  DParamMin=[]  DParamMax=[]  NParamMin=[]  NParamMax=[]  KbParamMin=[]  KbParamMax=[]  KtParamMin=[]  KtParamMax=[]  KbOutMin=[]  KbOutMax=[]  KtOutMin=[]  KtOutMax=[]  IntegratorOutMin=[]  IntegratorOutMax=[]  FilterOutMin=[]  FilterOutMax=[]  SumI1OutMin=[]  SumI1OutMax=[]  SumI2OutMin=[]  SumI2OutMax=[]  SumI3OutMin=[]  SumI3OutMax=[]  SumI4OutMin=[]  SumI4OutMax=[]  SumDOutMin=[]  SumDOutMax=[]  DifferentiatorOutMin=[]  DifferentiatorOutMax=[]  FilterDiffOutCoefMin=[]  FilterDiffOutCoefMax=[]  ReciprocalOutMin=[]  ReciprocalOutMax=[]  SumDenOutMin=[]  SumDenOutMax=[]  SumNumOutMin=[]  SumNumOutMax=[]  DivideOutMin=[]  DivideOutMax=[]  IntegratorContinuousStateAttributes=''  IntegratorStateMustResolveToSignalObject=off  IntegratorRTWStateStorageClass=Auto  FilterContinuousStateAttributes=''  FilterStateMustResolveToSignalObject=off  FilterRTWStateStorageClass=Auto  ParallelPVariant=InternalParameters  IdealPVariant=Disabled  IVariant=InternalParameters  DVariant=Disabled  IntegratorVariant=Discrete  SatVariant=Disabled  AWVariant=Passthrough  PCopyVariant=Disabled  TRVariant=Disabled  FdbkBlocksVariant=Forward  IdealPFdbkVariant=Disabled  SatFdbkVariant=Disabled  DerivativeFilterVariant=Disabled  NVariant=Disabled  NCopyVariant=Disabled_SignalSpec  FilterICVariant=Disabled  IntegratorICVariant=InternalICs  ExternalResetVariant=Disabled  TRSumVariant=Passthrough  SumFdbkVariant=Disabled  SumVariant=Sum_PI
  PID Controller4 : simulink/Continuous/PID Controller  Controller=PI  Form=Parallel  TimeDomain=Discrete-time  SampleTime=ts  IntegratorMethod=Forward Euler  FilterMethod=Forward Euler  ControllerParametersSource=internal  P=0.00659405389444924  I=0.324359106529765  D=0  UseFilter=on  N=0  TunerSelectOption=Transfer Function Based (PID Tuner App)  InitialConditionSource=internal  InitialConditionForIntegrator=0  InitialConditionForFilter=0  DifferentiatorICPrevScaledInput=0  ExternalReset=none  TrackingMode=off  Kt=1  LimitOutput=off  UpperSaturationLimit=0.001  LowerSaturationLimit=-0.001  LinearizeAsGain=on  AntiWindupMode=none  Kb=1  POutMin=[]  POutMax=[]  IOutMin=[]  IOutMax=[]  DOutMin=[]  DOutMax=[]  NOutMin=[]  NOutMax=[]  SumOutMin=[]  SumOutMax=[]  SaturationOutMin=[]  SaturationOutMax=[]  PParamMin=[]  PParamMax=[]  IParamMin=[]  IParamMax=[]  DParamMin=[]  DParamMax=[]  NParamMin=[]  NParamMax=[]  KbParamMin=[]  KbParamMax=[]  KtParamMin=[]  KtParamMax=[]  KbOutMin=[]  KbOutMax=[]  KtOutMin=[]  KtOutMax=[]  IntegratorOutMin=[]  IntegratorOutMax=[]  FilterOutMin=[]  FilterOutMax=[]  SumI1OutMin=[]  SumI1OutMax=[]  SumI2OutMin=[]  SumI2OutMax=[]  SumI3OutMin=[]  SumI3OutMax=[]  SumI4OutMin=[]  SumI4OutMax=[]  SumDOutMin=[]  SumDOutMax=[]  DifferentiatorOutMin=[]  DifferentiatorOutMax=[]  FilterDiffOutCoefMin=[]  FilterDiffOutCoefMax=[]  ReciprocalOutMin=[]  ReciprocalOutMax=[]  SumDenOutMin=[]  SumDenOutMax=[]  SumNumOutMin=[]  SumNumOutMax=[]  DivideOutMin=[]  DivideOutMax=[]  IntegratorContinuousStateAttributes=''  IntegratorStateMustResolveToSignalObject=off  IntegratorRTWStateStorageClass=Auto  FilterContinuousStateAttributes=''  FilterStateMustResolveToSignalObject=off  FilterRTWStateStorageClass=Auto  ParallelPVariant=InternalParameters  IdealPVariant=Disabled  IVariant=InternalParameters  DVariant=Disabled  IntegratorVariant=Discrete  SatVariant=Disabled  AWVariant=Passthrough  PCopyVariant=Disabled  TRVariant=Disabled  FdbkBlocksVariant=Forward  IdealPFdbkVariant=Disabled  SatFdbkVariant=Disabled  DerivativeFilterVariant=Disabled  NVariant=Disabled  NCopyVariant=Disabled_SignalSpec  FilterICVariant=Disabled  IntegratorICVariant=InternalICs  ExternalResetVariant=Disabled  TRSumVariant=Passthrough  SumFdbkVariant=Disabled  SumVariant=Sum_PI
  PID Controller5 : simulink/Continuous/PID Controller  Controller=PI  Form=Parallel  TimeDomain=Discrete-time  SampleTime=ts  IntegratorMethod=Forward Euler  FilterMethod=Forward Euler  ControllerParametersSource=internal  P=0.00683255135393729  I=0.146143607435002  D=0  UseFilter=on  N=0  TunerSelectOption=Transfer Function Based (PID Tuner App)  InitialConditionSource=internal  InitialConditionForIntegrator=0  InitialConditionForFilter=0  DifferentiatorICPrevScaledInput=0  ExternalReset=none  TrackingMode=off  Kt=1  LimitOutput=off  UpperSaturationLimit=0.001  LowerSaturationLimit=-0.001  LinearizeAsGain=on  AntiWindupMode=none  Kb=1  POutMin=[]  POutMax=[]  IOutMin=[]  IOutMax=[]  DOutMin=[]  DOutMax=[]  NOutMin=[]  NOutMax=[]  SumOutMin=[]  SumOutMax=[]  SaturationOutMin=[]  SaturationOutMax=[]  PParamMin=[]  PParamMax=[]  IParamMin=[]  IParamMax=[]  DParamMin=[]  DParamMax=[]  NParamMin=[]  NParamMax=[]  KbParamMin=[]  KbParamMax=[]  KtParamMin=[]  KtParamMax=[]  KbOutMin=[]  KbOutMax=[]  KtOutMin=[]  KtOutMax=[]  IntegratorOutMin=[]  IntegratorOutMax=[]  FilterOutMin=[]  FilterOutMax=[]  SumI1OutMin=[]  SumI1OutMax=[]  SumI2OutMin=[]  SumI2OutMax=[]  SumI3OutMin=[]  SumI3OutMax=[]  SumI4OutMin=[]  SumI4OutMax=[]  SumDOutMin=[]  SumDOutMax=[]  DifferentiatorOutMin=[]  DifferentiatorOutMax=[]  FilterDiffOutCoefMin=[]  FilterDiffOutCoefMax=[]  ReciprocalOutMin=[]  ReciprocalOutMax=[]  SumDenOutMin=[]  SumDenOutMax=[]  SumNumOutMin=[]  SumNumOutMax=[]  DivideOutMin=[]  DivideOutMax=[]  IntegratorContinuousStateAttributes=''  IntegratorStateMustResolveToSignalObject=off  IntegratorRTWStateStorageClass=Auto  FilterContinuousStateAttributes=''  FilterStateMustResolveToSignalObject=off  FilterRTWStateStorageClass=Auto  ParallelPVariant=InternalParameters  IdealPVariant=Disabled  IVariant=InternalParameters  DVariant=Disabled  IntegratorVariant=Discrete  SatVariant=Disabled  AWVariant=Passthrough  PCopyVariant=Disabled  TRVariant=Disabled  FdbkBlocksVariant=Forward  IdealPFdbkVariant=Disabled  SatFdbkVariant=Disabled  DerivativeFilterVariant=Disabled  NVariant=Disabled  NCopyVariant=Disabled_SignalSpec  FilterICVariant=Disabled  IntegratorICVariant=InternalICs  ExternalResetVariant=Disabled  TRSumVariant=Passthrough  SumFdbkVariant=Disabled  SumVariant=Sum_PI
  filter{,1..5} (6 alike) : controlLibrary/filter  tc=1e-2  sampleTime=ts
  tRef : Outport  OutDataTypeStr=Bus: jointTorqueBus  Unit=N*m
  wires:
  Gain13/1 -> [RFA_w]
  Gain4/1 -> [UA_w]
  Bus Selector1/6 -> Gain16/1  "<leftFingerJointVel>"
  Bus Selector/2 -> Gain3/1  "<foreArmJointVel>"
  [FA_tRef] -> Bus Creator2/2  "FAtRef"
  Gain10/1 -> [GA_w]
  [GA_tRef] -> Bus Creator2/4  "GAtRef"
  Bus Selector1/1 -> Gain4/1  "<upperArmJointVel>"
  Bus Selector/1 -> Gain2/1  "<upperArmJointVel>"
  Gain7/1 -> [WA_w]
  w/1 -> Bus Selector1/1
  Bus Selector/3 -> Gain6/1  "<wristJointVel>"
  Bus Selector1/3 -> Gain7/1  "<wristJointVel>"
  Bus Selector1/2 -> Gain5/1  "<foreArmJointVel>"
  wRef/1 -> Bus Selector/1
  Gain6/1 -> [WA_wRef]
  Gain15/1 -> [LFA_wRef]
  Gain5/1 -> [FA_w]
  Bus Selector/4 -> Gain9/1  "<gripperJointVel>"
  [WA_tRef] -> Bus Creator2/3  "WAtRef"
  Gain9/1 -> [GA_wRef]
  Gain16/1 -> [LFA_w]
  Gain12/1 -> [RFA_wRef]
  Bus Selector1/5 -> Gain13/1  "<rightFingerJointVel>"
  Bus Selector/6 -> Gain15/1  "<leftFingerJointVel>"
  Gain3/1 -> [FA_wRef]
  [RFA_tRef] -> Bus Creator2/5  "RFAtRef"
  Bus Selector/5 -> Gain12/1  "<rightFingerJointVel>"
  Bus Selector1/4 -> Gain10/1  "<gripperJointVel>"
  Gain2/1 -> [UA_wRef]
  [LFA_tRef] -> Bus Creator2/6  "LFAtRef"
  [UA_tRef] -> Bus Creator2/1  "UAtRef"
  Bus Creator2/1 -> tRef/1  "torqueReference"
  [GA_w] -> filter3/2
  [RFA_wRef] -> filter4/1
  [FA_w] -> filter1/2
  [WA_wRef] -> filter2/1
  PID Controller2/1 -> [WA_tRef]
  PID Controller5/1 -> [LFA_tRef]
  [LFA_wRef] -> filter5/1
  PID Controller3/1 -> [GA_tRef]
  [FA_wRef] -> filter1/1
  PID Controller4/1 -> [RFA_tRef]
  [LFA_w] -> filter5/2
  [GA_wRef] -> filter3/1
  [RFA_w] -> filter4/2
  [UA_w] -> filter/2
  [UA_wRef] -> filter/1
  [WA_w] -> filter2/2
  PID Controller/1 -> [UA_tRef]
  filter/1 -> PID Controller/1
  filter1/1 -> PID Controller1/1
  PID Controller1/1 -> [FA_tRef]
  filter2/1 -> PID Controller2/1
  filter3/1 -> PID Controller3/1
  filter4/1 -> PID Controller4/1
  filter5/1 -> PID Controller5/1
